simulink model "buckBoostConverter"  (R2022b)
settings: Solver=VariableStepAuto  StartTime=0.0  StopTime=10.0  RelTol=1e-3
undefined symbols (not defined in the file): k
settings Model: Creator=mithi  LastModifiedBy=mithi

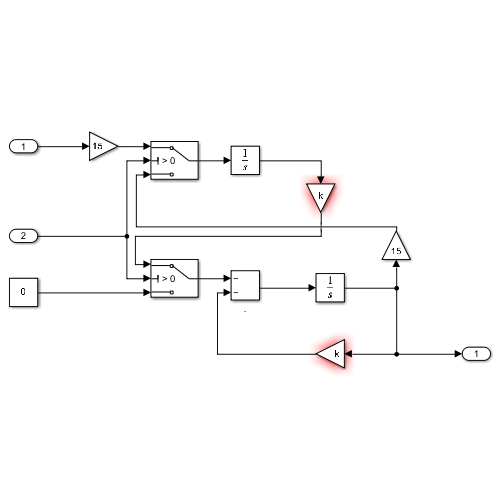
[thumbnail: Simulink's stored preview of the top-level diagram]
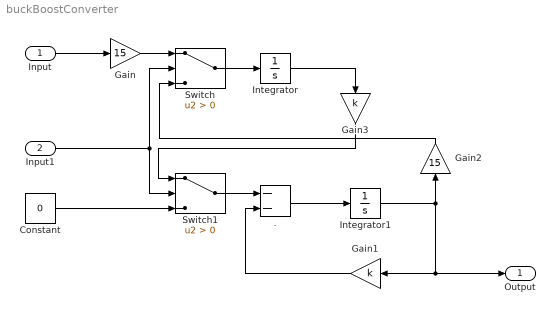
== system buckBoostConverter ==
  Input : Inport
  Input1 : Inport  Port=2
  . : Sum  Inputs=--
  Constant : Constant  Value=0
  Gain : Gain  Gain=15
  Gain1 : Gain  Gain=k
  Gain2 : Gain  Gain=15
  Gain3 : Gain  Gain=k
  Integrator : Integrator
  Integrator1 : Integrator
  Switch : Switch  Criteria=u2 > Threshold  SaturateOnIntegerOverflow=off  InputSameDT=off
  Switch1 : Switch  Criteria=u2 > Threshold  SaturateOnIntegerOverflow=off  InputSameDT=off
  Output : Outport
  wires:
  Input/1 -> Gain/1
  Gain/1 -> Switch/1
  Switch/1 -> Integrator/1
  Integrator/1 -> Gain3/1
  Gain3/1 -> Switch1/1
  Input1/1 -> Switch1/2, Switch/2
  Constant/1 -> Switch1/3
  Gain1/1 -> ./2
  Switch1/1 -> ./1
  ./1 -> Integrator1/1
  Integrator1/1 -> Gain2/1, Gain1/1, Output/1
  Gain2/1 -> Switch/3
